simulink model "gm_ZynqBF_2tx_fpga"  (R2018b)
settings: Solver=FixedStepDiscrete  StartTime=0.0  StopTime=10.0  FixedStep=(1/420e3)/128  RelTol=1e-3
undefined symbols (not defined in the file or in its folder): a, b, c
libraries: hdlsllib x873, simulink x349
(part 38 of 40)

== system gm_ZynqBF_2tx_fpga/channel_estimator/peakdetect_ch1/correlator1/rx_ram_q_instance21/get_bit ==
  u : Inport  OutDataTypeStr=fixdt(0, 64, 0)  PortDimensions=1  SampleTime=1.86011904761905e-08
  ind : Inport  Port=2  OutDataTypeStr=fixdt(0, 9, 0)  PortDimensions=1  SampleTime=1.86011904761905e-08
  get_bit : MATLAB Function  TreatAsAtomicUnit=on
  y : Outport
  wires:
  get_bit/1(y) -> y/1
  ind/1 -> get_bit/2(ind)
  u/1 -> get_bit/1(u)

== system gm_ZynqBF_2tx_fpga/channel_estimator/peakdetect_ch1/correlator1/rx_ram_q_instance22/get_bit ==
  u : Inport  OutDataTypeStr=fixdt(0, 64, 0)  PortDimensions=1  SampleTime=1.86011904761905e-08
  ind : Inport  Port=2  OutDataTypeStr=fixdt(0, 9, 0)  PortDimensions=1  SampleTime=1.86011904761905e-08
  get_bit : MATLAB Function  TreatAsAtomicUnit=on
  y : Outport
  wires:
  get_bit/1(y) -> y/1
  ind/1 -> get_bit/2(ind)
  u/1 -> get_bit/1(u)

== system gm_ZynqBF_2tx_fpga/channel_estimator/peakdetect_ch1/correlator1/rx_ram_q_instance23/get_bit ==
  u : Inport  OutDataTypeStr=fixdt(0, 64, 0)  PortDimensions=1  SampleTime=1.86011904761905e-08
  ind : Inport  Port=2  OutDataTypeStr=fixdt(0, 9, 0)  PortDimensions=1  SampleTime=1.86011904761905e-08
  get_bit : MATLAB Function  TreatAsAtomicUnit=on
  y : Outport
  wires:
  get_bit/1(y) -> y/1
  ind/1 -> get_bit/2(ind)
  u/1 -> get_bit/1(u)

== system gm_ZynqBF_2tx_fpga/channel_estimator/peakdetect_ch1/correlator1/rx_ram_q_instance24/get_bit ==
  u : Inport  OutDataTypeStr=fixdt(0, 64, 0)  PortDimensions=1  SampleTime=1.86011904761905e-08
  ind : Inport  Port=2  OutDataTypeStr=fixdt(0, 9, 0)  PortDimensions=1  SampleTime=1.86011904761905e-08
  get_bit : MATLAB Function  TreatAsAtomicUnit=on
  y : Outport
  wires:
  get_bit/1(y) -> y/1
  ind/1 -> get_bit/2(ind)
  u/1 -> get_bit/1(u)

== system gm_ZynqBF_2tx_fpga/channel_estimator/peakdetect_ch1/correlator1/rx_ram_q_instance25/get_bit ==
  u : Inport  OutDataTypeStr=fixdt(0, 64, 0)  PortDimensions=1  SampleTime=1.86011904761905e-08
  ind : Inport  Port=2  OutDataTypeStr=fixdt(0, 9, 0)  PortDimensions=1  SampleTime=1.86011904761905e-08
  get_bit : MATLAB Function  TreatAsAtomicUnit=on
  y : Outport
  wires:
  get_bit/1(y) -> y/1
  ind/1 -> get_bit/2(ind)
  u/1 -> get_bit/1(u)

== system gm_ZynqBF_2tx_fpga/channel_estimator/peakdetect_ch1/correlator1/rx_ram_q_instance26/get_bit ==
  u : Inport  OutDataTypeStr=fixdt(0, 64, 0)  PortDimensions=1  SampleTime=1.86011904761905e-08
  ind : Inport  Port=2  OutDataTypeStr=fixdt(0, 9, 0)  PortDimensions=1  SampleTime=1.86011904761905e-08
  get_bit : MATLAB Function  TreatAsAtomicUnit=on
  y : Outport
  wires:
  get_bit/1(y) -> y/1
  ind/1 -> get_bit/2(ind)
  u/1 -> get_bit/1(u)

== system gm_ZynqBF_2tx_fpga/channel_estimator/peakdetect_ch1/correlator1/rx_ram_q_instance27/get_bit ==
  u : Inport  OutDataTypeStr=fixdt(0, 64, 0)  PortDimensions=1  SampleTime=1.86011904761905e-08
  ind : Inport  Port=2  OutDataTypeStr=fixdt(0, 9, 0)  PortDimensions=1  SampleTime=1.86011904761905e-08
  get_bit : MATLAB Function  TreatAsAtomicUnit=on
  y : Outport
  wires:
  get_bit/1(y) -> y/1
  ind/1 -> get_bit/2(ind)
  u/1 -> get_bit/1(u)

== system gm_ZynqBF_2tx_fpga/channel_estimator/peakdetect_ch1/correlator1/rx_ram_q_instance28/get_bit ==
  u : Inport  OutDataTypeStr=fixdt(0, 64, 0)  PortDimensions=1  SampleTime=1.86011904761905e-08
  ind : Inport  Port=2  OutDataTypeStr=fixdt(0, 9, 0)  PortDimensions=1  SampleTime=1.86011904761905e-08
  get_bit : MATLAB Function  TreatAsAtomicUnit=on
  y : Outport
  wires:
  get_bit/1(y) -> y/1
  ind/1 -> get_bit/2(ind)
  u/1 -> get_bit/1(u)

== system gm_ZynqBF_2tx_fpga/channel_estimator/peakdetect_ch1/correlator1/rx_ram_q_instance29/get_bit ==
  u : Inport  OutDataTypeStr=fixdt(0, 64, 0)  PortDimensions=1  SampleTime=1.86011904761905e-08
  ind : Inport  Port=2  OutDataTypeStr=fixdt(0, 9, 0)  PortDimensions=1  SampleTime=1.86011904761905e-08
  get_bit : MATLAB Function  TreatAsAtomicUnit=on
  y : Outport
  wires:
  get_bit/1(y) -> y/1
  ind/1 -> get_bit/2(ind)
  u/1 -> get_bit/1(u)

== system gm_ZynqBF_2tx_fpga/channel_estimator/peakdetect_ch1/correlator1/rx_ram_q_instance3/get_bit ==
  u : Inport  OutDataTypeStr=fixdt(0, 64, 0)  PortDimensions=1  SampleTime=1.86011904761905e-08
  ind : Inport  Port=2  OutDataTypeStr=fixdt(0, 9, 0)  PortDimensions=1  SampleTime=1.86011904761905e-08
  get_bit : MATLAB Function  TreatAsAtomicUnit=on
  y : Outport
  wires:
  get_bit/1(y) -> y/1
  ind/1 -> get_bit/2(ind)
  u/1 -> get_bit/1(u)

== system gm_ZynqBF_2tx_fpga/channel_estimator/peakdetect_ch1/correlator1/rx_ram_q_instance30/get_bit ==
  u : Inport  OutDataTypeStr=fixdt(0, 64, 0)  PortDimensions=1  SampleTime=1.86011904761905e-08
  ind : Inport  Port=2  OutDataTypeStr=fixdt(0, 9, 0)  PortDimensions=1  SampleTime=1.86011904761905e-08
  get_bit : MATLAB Function  TreatAsAtomicUnit=on
  y : Outport
  wires:
  get_bit/1(y) -> y/1
  ind/1 -> get_bit/2(ind)
  u/1 -> get_bit/1(u)

== system gm_ZynqBF_2tx_fpga/channel_estimator/peakdetect_ch1/correlator1/rx_ram_q_instance31/get_bit ==
  u : Inport  OutDataTypeStr=fixdt(0, 64, 0)  PortDimensions=1  SampleTime=1.86011904761905e-08
  ind : Inport  Port=2  OutDataTypeStr=fixdt(0, 9, 0)  PortDimensions=1  SampleTime=1.86011904761905e-08
  get_bit : MATLAB Function  TreatAsAtomicUnit=on
  y : Outport
  wires:
  get_bit/1(y) -> y/1
  ind/1 -> get_bit/2(ind)
  u/1 -> get_bit/1(u)

== system gm_ZynqBF_2tx_fpga/channel_estimator/peakdetect_ch1/correlator1/rx_ram_q_instance32/get_bit ==
  u : Inport  OutDataTypeStr=fixdt(0, 64, 0)  PortDimensions=1  SampleTime=1.86011904761905e-08
  ind : Inport  Port=2  OutDataTypeStr=fixdt(0, 9, 0)  PortDimensions=1  SampleTime=1.86011904761905e-08
  get_bit : MATLAB Function  TreatAsAtomicUnit=on
  y : Outport
  wires:
  get_bit/1(y) -> y/1
  ind/1 -> get_bit/2(ind)
  u/1 -> get_bit/1(u)

== system gm_ZynqBF_2tx_fpga/channel_estimator/peakdetect_ch1/correlator1/rx_ram_q_instance33/get_bit ==
  u : Inport  OutDataTypeStr=fixdt(0, 64, 0)  PortDimensions=1  SampleTime=1.86011904761905e-08
  ind : Inport  Port=2  OutDataTypeStr=fixdt(0, 9, 0)  PortDimensions=1  SampleTime=1.86011904761905e-08
  get_bit : MATLAB Function  TreatAsAtomicUnit=on
  y : Outport
  wires:
  get_bit/1(y) -> y/1
  ind/1 -> get_bit/2(ind)
  u/1 -> get_bit/1(u)

== system gm_ZynqBF_2tx_fpga/channel_estimator/peakdetect_ch1/correlator1/rx_ram_q_instance34/get_bit ==
  u : Inport  OutDataTypeStr=fixdt(0, 64, 0)  PortDimensions=1  SampleTime=1.86011904761905e-08
  ind : Inport  Port=2  OutDataTypeStr=fixdt(0, 9, 0)  PortDimensions=1  SampleTime=1.86011904761905e-08
  get_bit : MATLAB Function  TreatAsAtomicUnit=on
  y : Outport
  wires:
  get_bit/1(y) -> y/1
  ind/1 -> get_bit/2(ind)
  u/1 -> get_bit/1(u)

== system gm_ZynqBF_2tx_fpga/channel_estimator/peakdetect_ch1/correlator1/rx_ram_q_instance35/get_bit ==
  u : Inport  OutDataTypeStr=fixdt(0, 64, 0)  PortDimensions=1  SampleTime=1.86011904761905e-08
  ind : Inport  Port=2  OutDataTypeStr=fixdt(0, 9, 0)  PortDimensions=1  SampleTime=1.86011904761905e-08
  get_bit : MATLAB Function  TreatAsAtomicUnit=on
  y : Outport
  wires:
  get_bit/1(y) -> y/1
  ind/1 -> get_bit/2(ind)
  u/1 -> get_bit/1(u)

== system gm_ZynqBF_2tx_fpga/channel_estimator/peakdetect_ch1/correlator1/rx_ram_q_instance36/get_bit ==
  u : Inport  OutDataTypeStr=fixdt(0, 64, 0)  PortDimensions=1  SampleTime=1.86011904761905e-08
  ind : Inport  Port=2  OutDataTypeStr=fixdt(0, 9, 0)  PortDimensions=1  SampleTime=1.86011904761905e-08
  get_bit : MATLAB Function  TreatAsAtomicUnit=on
  y : Outport
  wires:
  get_bit/1(y) -> y/1
  ind/1 -> get_bit/2(ind)
  u/1 -> get_bit/1(u)

== system gm_ZynqBF_2tx_fpga/channel_estimator/peakdetect_ch1/correlator1/rx_ram_q_instance37/get_bit ==
  u : Inport  OutDataTypeStr=fixdt(0, 64, 0)  PortDimensions=1  SampleTime=1.86011904761905e-08
  ind : Inport  Port=2  OutDataTypeStr=fixdt(0, 9, 0)  PortDimensions=1  SampleTime=1.86011904761905e-08
  get_bit : MATLAB Function  TreatAsAtomicUnit=on
  y : Outport
  wires:
  get_bit/1(y) -> y/1
  ind/1 -> get_bit/2(ind)
  u/1 -> get_bit/1(u)

== system gm_ZynqBF_2tx_fpga/channel_estimator/peakdetect_ch1/correlator1/rx_ram_q_instance38/get_bit ==
  u : Inport  OutDataTypeStr=fixdt(0, 64, 0)  PortDimensions=1  SampleTime=1.86011904761905e-08
  ind : Inport  Port=2  OutDataTypeStr=fixdt(0, 9, 0)  PortDimensions=1  SampleTime=1.86011904761905e-08
  get_bit : MATLAB Function  TreatAsAtomicUnit=on
  y : Outport
  wires:
  get_bit/1(y) -> y/1
  ind/1 -> get_bit/2(ind)
  u/1 -> get_bit/1(u)

== system gm_ZynqBF_2tx_fpga/channel_estimator/peakdetect_ch1/correlator1/rx_ram_q_instance39/get_bit ==
  u : Inport  OutDataTypeStr=fixdt(0, 64, 0)  PortDimensions=1  SampleTime=1.86011904761905e-08
  ind : Inport  Port=2  OutDataTypeStr=fixdt(0, 9, 0)  PortDimensions=1  SampleTime=1.86011904761905e-08
  get_bit : MATLAB Function  TreatAsAtomicUnit=on
  y : Outport
  wires:
  get_bit/1(y) -> y/1
  ind/1 -> get_bit/2(ind)
  u/1 -> get_bit/1(u)

== system gm_ZynqBF_2tx_fpga/channel_estimator/peakdetect_ch1/correlator1/rx_ram_q_instance4/get_bit ==
  u : Inport  OutDataTypeStr=fixdt(0, 64, 0)  PortDimensions=1  SampleTime=1.86011904761905e-08
  ind : Inport  Port=2  OutDataTypeStr=fixdt(0, 9, 0)  PortDimensions=1  SampleTime=1.86011904761905e-08
  get_bit : MATLAB Function  TreatAsAtomicUnit=on
  y : Outport
  wires:
  get_bit/1(y) -> y/1
  ind/1 -> get_bit/2(ind)
  u/1 -> get_bit/1(u)

== system gm_ZynqBF_2tx_fpga/channel_estimator/peakdetect_ch1/correlator1/rx_ram_q_instance40/get_bit ==
  u : Inport  OutDataTypeStr=fixdt(0, 64, 0)  PortDimensions=1  SampleTime=1.86011904761905e-08
  ind : Inport  Port=2  OutDataTypeStr=fixdt(0, 9, 0)  PortDimensions=1  SampleTime=1.86011904761905e-08
  get_bit : MATLAB Function  TreatAsAtomicUnit=on
  y : Outport
  wires:
  get_bit/1(y) -> y/1
  ind/1 -> get_bit/2(ind)
  u/1 -> get_bit/1(u)

== system gm_ZynqBF_2tx_fpga/channel_estimator/peakdetect_ch1/correlator1/rx_ram_q_instance41/get_bit ==
  u : Inport  OutDataTypeStr=fixdt(0, 64, 0)  PortDimensions=1  SampleTime=1.86011904761905e-08
  ind : Inport  Port=2  OutDataTypeStr=fixdt(0, 9, 0)  PortDimensions=1  SampleTime=1.86011904761905e-08
  get_bit : MATLAB Function  TreatAsAtomicUnit=on
  y : Outport
  wires:
  get_bit/1(y) -> y/1
  ind/1 -> get_bit/2(ind)
  u/1 -> get_bit/1(u)

== system gm_ZynqBF_2tx_fpga/channel_estimator/peakdetect_ch1/correlator1/rx_ram_q_instance42/get_bit ==
  u : Inport  OutDataTypeStr=fixdt(0, 64, 0)  PortDimensions=1  SampleTime=1.86011904761905e-08
  ind : Inport  Port=2  OutDataTypeStr=fixdt(0, 9, 0)  PortDimensions=1  SampleTime=1.86011904761905e-08
  get_bit : MATLAB Function  TreatAsAtomicUnit=on
  y : Outport
  wires:
  get_bit/1(y) -> y/1
  ind/1 -> get_bit/2(ind)
  u/1 -> get_bit/1(u)

== system gm_ZynqBF_2tx_fpga/channel_estimator/peakdetect_ch1/correlator1/rx_ram_q_instance43/get_bit ==
  u : Inport  OutDataTypeStr=fixdt(0, 64, 0)  PortDimensions=1  SampleTime=1.86011904761905e-08
  ind : Inport  Port=2  OutDataTypeStr=fixdt(0, 9, 0)  PortDimensions=1  SampleTime=1.86011904761905e-08
  get_bit : MATLAB Function  TreatAsAtomicUnit=on
  y : Outport
  wires:
  get_bit/1(y) -> y/1
  ind/1 -> get_bit/2(ind)
  u/1 -> get_bit/1(u)

== system gm_ZynqBF_2tx_fpga/channel_estimator/peakdetect_ch1/correlator1/rx_ram_q_instance44/get_bit ==
  u : Inport  OutDataTypeStr=fixdt(0, 64, 0)  PortDimensions=1  SampleTime=1.86011904761905e-08
  ind : Inport  Port=2  OutDataTypeStr=fixdt(0, 9, 0)  PortDimensions=1  SampleTime=1.86011904761905e-08
  get_bit : MATLAB Function  TreatAsAtomicUnit=on
  y : Outport
  wires:
  get_bit/1(y) -> y/1
  ind/1 -> get_bit/2(ind)
  u/1 -> get_bit/1(u)

== system gm_ZynqBF_2tx_fpga/channel_estimator/peakdetect_ch1/correlator1/rx_ram_q_instance45/get_bit ==
  u : Inport  OutDataTypeStr=fixdt(0, 64, 0)  PortDimensions=1  SampleTime=1.86011904761905e-08
  ind : Inport  Port=2  OutDataTypeStr=fixdt(0, 9, 0)  PortDimensions=1  SampleTime=1.86011904761905e-08
  get_bit : MATLAB Function  TreatAsAtomicUnit=on
  y : Outport
  wires:
  get_bit/1(y) -> y/1
  ind/1 -> get_bit/2(ind)
  u/1 -> get_bit/1(u)

== system gm_ZynqBF_2tx_fpga/channel_estimator/peakdetect_ch1/correlator1/rx_ram_q_instance46/get_bit ==
  u : Inport  OutDataTypeStr=fixdt(0, 64, 0)  PortDimensions=1  SampleTime=1.86011904761905e-08
  ind : Inport  Port=2  OutDataTypeStr=fixdt(0, 9, 0)  PortDimensions=1  SampleTime=1.86011904761905e-08
  get_bit : MATLAB Function  TreatAsAtomicUnit=on
  y : Outport
  wires:
  get_bit/1(y) -> y/1
  ind/1 -> get_bit/2(ind)
  u/1 -> get_bit/1(u)

== system gm_ZynqBF_2tx_fpga/channel_estimator/peakdetect_ch1/correlator1/rx_ram_q_instance47/get_bit ==
  u : Inport  OutDataTypeStr=fixdt(0, 64, 0)  PortDimensions=1  SampleTime=1.86011904761905e-08
  ind : Inport  Port=2  OutDataTypeStr=fixdt(0, 9, 0)  PortDimensions=1  SampleTime=1.86011904761905e-08
  get_bit : MATLAB Function  TreatAsAtomicUnit=on
  y : Outport
  wires:
  get_bit/1(y) -> y/1
  ind/1 -> get_bit/2(ind)
  u/1 -> get_bit/1(u)

== system gm_ZynqBF_2tx_fpga/channel_estimator/peakdetect_ch1/correlator1/rx_ram_q_instance48/get_bit ==
  u : Inport  OutDataTypeStr=fixdt(0, 64, 0)  PortDimensions=1  SampleTime=1.86011904761905e-08
  ind : Inport  Port=2  OutDataTypeStr=fixdt(0, 9, 0)  PortDimensions=1  SampleTime=1.86011904761905e-08
  get_bit : MATLAB Function  TreatAsAtomicUnit=on
  y : Outport
  wires:
  get_bit/1(y) -> y/1
  ind/1 -> get_bit/2(ind)
  u/1 -> get_bit/1(u)

== system gm_ZynqBF_2tx_fpga/channel_estimator/peakdetect_ch1/correlator1/rx_ram_q_instance49/get_bit ==
  u : Inport  OutDataTypeStr=fixdt(0, 64, 0)  PortDimensions=1  SampleTime=1.86011904761905e-08
  ind : Inport  Port=2  OutDataTypeStr=fixdt(0, 9, 0)  PortDimensions=1  SampleTime=1.86011904761905e-08
  get_bit : MATLAB Function  TreatAsAtomicUnit=on
  y : Outport
  wires:
  get_bit/1(y) -> y/1
  ind/1 -> get_bit/2(ind)
  u/1 -> get_bit/1(u)

== system gm_ZynqBF_2tx_fpga/channel_estimator/peakdetect_ch1/correlator1/rx_ram_q_instance5/get_bit ==
  u : Inport  OutDataTypeStr=fixdt(0, 64, 0)  PortDimensions=1  SampleTime=1.86011904761905e-08
  ind : Inport  Port=2  OutDataTypeStr=fixdt(0, 9, 0)  PortDimensions=1  SampleTime=1.86011904761905e-08
  get_bit : MATLAB Function  TreatAsAtomicUnit=on
  y : Outport
  wires:
  get_bit/1(y) -> y/1
  ind/1 -> get_bit/2(ind)
  u/1 -> get_bit/1(u)

== system gm_ZynqBF_2tx_fpga/channel_estimator/peakdetect_ch1/correlator1/rx_ram_q_instance50/get_bit ==
  u : Inport  OutDataTypeStr=fixdt(0, 64, 0)  PortDimensions=1  SampleTime=1.86011904761905e-08
  ind : Inport  Port=2  OutDataTypeStr=fixdt(0, 9, 0)  PortDimensions=1  SampleTime=1.86011904761905e-08
  get_bit : MATLAB Function  TreatAsAtomicUnit=on
  y : Outport
  wires:
  get_bit/1(y) -> y/1
  ind/1 -> get_bit/2(ind)
  u/1 -> get_bit/1(u)

== system gm_ZynqBF_2tx_fpga/channel_estimator/peakdetect_ch1/correlator1/rx_ram_q_instance51/get_bit ==
  u : Inport  OutDataTypeStr=fixdt(0, 64, 0)  PortDimensions=1  SampleTime=1.86011904761905e-08
  ind : Inport  Port=2  OutDataTypeStr=fixdt(0, 9, 0)  PortDimensions=1  SampleTime=1.86011904761905e-08
  get_bit : MATLAB Function  TreatAsAtomicUnit=on
  y : Outport
  wires:
  get_bit/1(y) -> y/1
  ind/1 -> get_bit/2(ind)
  u/1 -> get_bit/1(u)

== system gm_ZynqBF_2tx_fpga/channel_estimator/peakdetect_ch1/correlator1/rx_ram_q_instance52/get_bit ==
  u : Inport  OutDataTypeStr=fixdt(0, 64, 0)  PortDimensions=1  SampleTime=1.86011904761905e-08
  ind : Inport  Port=2  OutDataTypeStr=fixdt(0, 9, 0)  PortDimensions=1  SampleTime=1.86011904761905e-08
  get_bit : MATLAB Function  TreatAsAtomicUnit=on
  y : Outport
  wires:
  get_bit/1(y) -> y/1
  ind/1 -> get_bit/2(ind)
  u/1 -> get_bit/1(u)

== system gm_ZynqBF_2tx_fpga/channel_estimator/peakdetect_ch1/correlator1/rx_ram_q_instance53/get_bit ==
  u : Inport  OutDataTypeStr=fixdt(0, 64, 0)  PortDimensions=1  SampleTime=1.86011904761905e-08
  ind : Inport  Port=2  OutDataTypeStr=fixdt(0, 9, 0)  PortDimensions=1  SampleTime=1.86011904761905e-08
  get_bit : MATLAB Function  TreatAsAtomicUnit=on
  y : Outport
  wires:
  get_bit/1(y) -> y/1
  ind/1 -> get_bit/2(ind)
  u/1 -> get_bit/1(u)

== system gm_ZynqBF_2tx_fpga/channel_estimator/peakdetect_ch1/correlator1/rx_ram_q_instance54/get_bit ==
  u : Inport  OutDataTypeStr=fixdt(0, 64, 0)  PortDimensions=1  SampleTime=1.86011904761905e-08
  ind : Inport  Port=2  OutDataTypeStr=fixdt(0, 9, 0)  PortDimensions=1  SampleTime=1.86011904761905e-08
  get_bit : MATLAB Function  TreatAsAtomicUnit=on
  y : Outport
  wires:
  get_bit/1(y) -> y/1
  ind/1 -> get_bit/2(ind)
  u/1 -> get_bit/1(u)

== system gm_ZynqBF_2tx_fpga/channel_estimator/peakdetect_ch1/correlator1/rx_ram_q_instance55/get_bit ==
  u : Inport  OutDataTypeStr=fixdt(0, 64, 0)  PortDimensions=1  SampleTime=1.86011904761905e-08
  ind : Inport  Port=2  OutDataTypeStr=fixdt(0, 9, 0)  PortDimensions=1  SampleTime=1.86011904761905e-08
  get_bit : MATLAB Function  TreatAsAtomicUnit=on
  y : Outport
  wires:
  get_bit/1(y) -> y/1
  ind/1 -> get_bit/2(ind)
  u/1 -> get_bit/1(u)

== system gm_ZynqBF_2tx_fpga/channel_estimator/peakdetect_ch1/correlator1/rx_ram_q_instance56/get_bit ==
  u : Inport  OutDataTypeStr=fixdt(0, 64, 0)  PortDimensions=1  SampleTime=1.86011904761905e-08
  ind : Inport  Port=2  OutDataTypeStr=fixdt(0, 9, 0)  PortDimensions=1  SampleTime=1.86011904761905e-08
  get_bit : MATLAB Function  TreatAsAtomicUnit=on
  y : Outport
  wires:
  get_bit/1(y) -> y/1
  ind/1 -> get_bit/2(ind)
  u/1 -> get_bit/1(u)

== system gm_ZynqBF_2tx_fpga/channel_estimator/peakdetect_ch1/correlator1/rx_ram_q_instance57/get_bit ==
  u : Inport  OutDataTypeStr=fixdt(0, 64, 0)  PortDimensions=1  SampleTime=1.86011904761905e-08
  ind : Inport  Port=2  OutDataTypeStr=fixdt(0, 9, 0)  PortDimensions=1  SampleTime=1.86011904761905e-08
  get_bit : MATLAB Function  TreatAsAtomicUnit=on
  y : Outport
  wires:
  get_bit/1(y) -> y/1
  ind/1 -> get_bit/2(ind)
  u/1 -> get_bit/1(u)

== system gm_ZynqBF_2tx_fpga/channel_estimator/peakdetect_ch1/correlator1/rx_ram_q_instance58/get_bit ==
  u : Inport  OutDataTypeStr=fixdt(0, 64, 0)  PortDimensions=1  SampleTime=1.86011904761905e-08
  ind : Inport  Port=2  OutDataTypeStr=fixdt(0, 9, 0)  PortDimensions=1  SampleTime=1.86011904761905e-08
  get_bit : MATLAB Function  TreatAsAtomicUnit=on
  y : Outport
  wires:
  get_bit/1(y) -> y/1
  ind/1 -> get_bit/2(ind)
  u/1 -> get_bit/1(u)

== system gm_ZynqBF_2tx_fpga/channel_estimator/peakdetect_ch1/correlator1/rx_ram_q_instance59/get_bit ==
  u : Inport  OutDataTypeStr=fixdt(0, 64, 0)  PortDimensions=1  SampleTime=1.86011904761905e-08
  ind : Inport  Port=2  OutDataTypeStr=fixdt(0, 9, 0)  PortDimensions=1  SampleTime=1.86011904761905e-08
  get_bit : MATLAB Function  TreatAsAtomicUnit=on
  y : Outport
  wires:
  get_bit/1(y) -> y/1
  ind/1 -> get_bit/2(ind)
  u/1 -> get_bit/1(u)

== system gm_ZynqBF_2tx_fpga/channel_estimator/peakdetect_ch1/correlator1/rx_ram_q_instance6/get_bit ==
  u : Inport  OutDataTypeStr=fixdt(0, 64, 0)  PortDimensions=1  SampleTime=1.86011904761905e-08
  ind : Inport  Port=2  OutDataTypeStr=fixdt(0, 9, 0)  PortDimensions=1  SampleTime=1.86011904761905e-08
  get_bit : MATLAB Function  TreatAsAtomicUnit=on
  y : Outport
  wires:
  get_bit/1(y) -> y/1
  ind/1 -> get_bit/2(ind)
  u/1 -> get_bit/1(u)

== system gm_ZynqBF_2tx_fpga/channel_estimator/peakdetect_ch1/correlator1/rx_ram_q_instance60/get_bit ==
  u : Inport  OutDataTypeStr=fixdt(0, 64, 0)  PortDimensions=1  SampleTime=1.86011904761905e-08
  ind : Inport  Port=2  OutDataTypeStr=fixdt(0, 9, 0)  PortDimensions=1  SampleTime=1.86011904761905e-08
  get_bit : MATLAB Function  TreatAsAtomicUnit=on
  y : Outport
  wires:
  get_bit/1(y) -> y/1
  ind/1 -> get_bit/2(ind)
  u/1 -> get_bit/1(u)

== system gm_ZynqBF_2tx_fpga/channel_estimator/peakdetect_ch1/correlator1/rx_ram_q_instance61/get_bit ==
  u : Inport  OutDataTypeStr=fixdt(0, 64, 0)  PortDimensions=1  SampleTime=1.86011904761905e-08
  ind : Inport  Port=2  OutDataTypeStr=fixdt(0, 9, 0)  PortDimensions=1  SampleTime=1.86011904761905e-08
  get_bit : MATLAB Function  TreatAsAtomicUnit=on
  y : Outport
  wires:
  get_bit/1(y) -> y/1
  ind/1 -> get_bit/2(ind)
  u/1 -> get_bit/1(u)

== system gm_ZynqBF_2tx_fpga/channel_estimator/peakdetect_ch1/correlator1/rx_ram_q_instance62/get_bit ==
  u : Inport  OutDataTypeStr=fixdt(0, 64, 0)  PortDimensions=1  SampleTime=1.86011904761905e-08
  ind : Inport  Port=2  OutDataTypeStr=fixdt(0, 9, 0)  PortDimensions=1  SampleTime=1.86011904761905e-08
  get_bit : MATLAB Function  TreatAsAtomicUnit=on
  y : Outport
  wires:
  get_bit/1(y) -> y/1
  ind/1 -> get_bit/2(ind)
  u/1 -> get_bit/1(u)

== system gm_ZynqBF_2tx_fpga/channel_estimator/peakdetect_ch1/correlator1/rx_ram_q_instance63/get_bit ==
  u : Inport  OutDataTypeStr=fixdt(0, 64, 0)  PortDimensions=1  SampleTime=1.86011904761905e-08
  ind : Inport  Port=2  OutDataTypeStr=fixdt(0, 9, 0)  PortDimensions=1  SampleTime=1.86011904761905e-08
  get_bit : MATLAB Function  TreatAsAtomicUnit=on
  y : Outport
  wires:
  get_bit/1(y) -> y/1
  ind/1 -> get_bit/2(ind)
  u/1 -> get_bit/1(u)

== system gm_ZynqBF_2tx_fpga/channel_estimator/peakdetect_ch1/correlator1/rx_ram_q_instance64/get_bit ==
  u : Inport  OutDataTypeStr=fixdt(0, 64, 0)  PortDimensions=1  SampleTime=1.86011904761905e-08
  ind : Inport  Port=2  OutDataTypeStr=fixdt(0, 9, 0)  PortDimensions=1  SampleTime=1.86011904761905e-08
  get_bit : MATLAB Function  TreatAsAtomicUnit=on
  y : Outport
  wires:
  get_bit/1(y) -> y/1
  ind/1 -> get_bit/2(ind)
  u/1 -> get_bit/1(u)

== system gm_ZynqBF_2tx_fpga/channel_estimator/peakdetect_ch1/correlator1/rx_ram_q_instance7/get_bit ==
  u : Inport  OutDataTypeStr=fixdt(0, 64, 0)  PortDimensions=1  SampleTime=1.86011904761905e-08
  ind : Inport  Port=2  OutDataTypeStr=fixdt(0, 9, 0)  PortDimensions=1  SampleTime=1.86011904761905e-08
  get_bit : MATLAB Function  TreatAsAtomicUnit=on
  y : Outport
  wires:
  get_bit/1(y) -> y/1
  ind/1 -> get_bit/2(ind)
  u/1 -> get_bit/1(u)

== system gm_ZynqBF_2tx_fpga/channel_estimator/peakdetect_ch1/correlator1/rx_ram_q_instance8/get_bit ==
  u : Inport  OutDataTypeStr=fixdt(0, 64, 0)  PortDimensions=1  SampleTime=1.86011904761905e-08
  ind : Inport  Port=2  OutDataTypeStr=fixdt(0, 9, 0)  PortDimensions=1  SampleTime=1.86011904761905e-08
  get_bit : MATLAB Function  TreatAsAtomicUnit=on
  y : Outport
  wires:
  get_bit/1(y) -> y/1
  ind/1 -> get_bit/2(ind)
  u/1 -> get_bit/1(u)

== system gm_ZynqBF_2tx_fpga/channel_estimator/peakdetect_ch1/correlator1/rx_ram_q_instance9/get_bit ==
  u : Inport  OutDataTypeStr=fixdt(0, 64, 0)  PortDimensions=1  SampleTime=1.86011904761905e-08
  ind : Inport  Port=2  OutDataTypeStr=fixdt(0, 9, 0)  PortDimensions=1  SampleTime=1.86011904761905e-08
  get_bit : MATLAB Function  TreatAsAtomicUnit=on
  y : Outport
  wires:
  get_bit/1(y) -> y/1
  ind/1 -> get_bit/2(ind)
  u/1 -> get_bit/1(u)

== system gm_ZynqBF_2tx_fpga/channel_estimator/peakdetect_ch2/correlator2/rx_ram_i_instance1/get_bit ==
  u : Inport  OutDataTypeStr=fixdt(0, 64, 0)  PortDimensions=1  SampleTime=1.86011904761905e-08
  ind : Inport  Port=2  OutDataTypeStr=fixdt(0, 9, 0)  PortDimensions=1  SampleTime=1.86011904761905e-08
  get_bit : MATLAB Function  TreatAsAtomicUnit=on
  y : Outport
  wires:
  get_bit/1(y) -> y/1
  ind/1 -> get_bit/2(ind)
  u/1 -> get_bit/1(u)

== system gm_ZynqBF_2tx_fpga/channel_estimator/peakdetect_ch2/correlator2/rx_ram_i_instance10/get_bit ==
  u : Inport  OutDataTypeStr=fixdt(0, 64, 0)  PortDimensions=1  SampleTime=1.86011904761905e-08
  ind : Inport  Port=2  OutDataTypeStr=fixdt(0, 9, 0)  PortDimensions=1  SampleTime=1.86011904761905e-08
  get_bit : MATLAB Function  TreatAsAtomicUnit=on
  y : Outport
  wires:
  get_bit/1(y) -> y/1
  ind/1 -> get_bit/2(ind)
  u/1 -> get_bit/1(u)

== system gm_ZynqBF_2tx_fpga/channel_estimator/peakdetect_ch2/correlator2/rx_ram_i_instance11/get_bit ==
  u : Inport  OutDataTypeStr=fixdt(0, 64, 0)  PortDimensions=1  SampleTime=1.86011904761905e-08
  ind : Inport  Port=2  OutDataTypeStr=fixdt(0, 9, 0)  PortDimensions=1  SampleTime=1.86011904761905e-08
  get_bit : MATLAB Function  TreatAsAtomicUnit=on
  y : Outport
  wires:
  get_bit/1(y) -> y/1
  ind/1 -> get_bit/2(ind)
  u/1 -> get_bit/1(u)

== system gm_ZynqBF_2tx_fpga/channel_estimator/peakdetect_ch2/correlator2/rx_ram_i_instance12/get_bit ==
  u : Inport  OutDataTypeStr=fixdt(0, 64, 0)  PortDimensions=1  SampleTime=1.86011904761905e-08
  ind : Inport  Port=2  OutDataTypeStr=fixdt(0, 9, 0)  PortDimensions=1  SampleTime=1.86011904761905e-08
  get_bit : MATLAB Function  TreatAsAtomicUnit=on
  y : Outport
  wires:
  get_bit/1(y) -> y/1
  ind/1 -> get_bit/2(ind)
  u/1 -> get_bit/1(u)

== system gm_ZynqBF_2tx_fpga/channel_estimator/peakdetect_ch2/correlator2/rx_ram_i_instance13/get_bit ==
  u : Inport  OutDataTypeStr=fixdt(0, 64, 0)  PortDimensions=1  SampleTime=1.86011904761905e-08
  ind : Inport  Port=2  OutDataTypeStr=fixdt(0, 9, 0)  PortDimensions=1  SampleTime=1.86011904761905e-08
  get_bit : MATLAB Function  TreatAsAtomicUnit=on
  y : Outport
  wires:
  get_bit/1(y) -> y/1
  ind/1 -> get_bit/2(ind)
  u/1 -> get_bit/1(u)

== system gm_ZynqBF_2tx_fpga/channel_estimator/peakdetect_ch2/correlator2/rx_ram_i_instance14/get_bit ==
  u : Inport  OutDataTypeStr=fixdt(0, 64, 0)  PortDimensions=1  SampleTime=1.86011904761905e-08
  ind : Inport  Port=2  OutDataTypeStr=fixdt(0, 9, 0)  PortDimensions=1  SampleTime=1.86011904761905e-08
  get_bit : MATLAB Function  TreatAsAtomicUnit=on
  y : Outport
  wires:
  get_bit/1(y) -> y/1
  ind/1 -> get_bit/2(ind)
  u/1 -> get_bit/1(u)

== system gm_ZynqBF_2tx_fpga/channel_estimator/peakdetect_ch2/correlator2/rx_ram_i_instance15/get_bit ==
  u : Inport  OutDataTypeStr=fixdt(0, 64, 0)  PortDimensions=1  SampleTime=1.86011904761905e-08
  ind : Inport  Port=2  OutDataTypeStr=fixdt(0, 9, 0)  PortDimensions=1  SampleTime=1.86011904761905e-08
  get_bit : MATLAB Function  TreatAsAtomicUnit=on
  y : Outport
  wires:
  get_bit/1(y) -> y/1
  ind/1 -> get_bit/2(ind)
  u/1 -> get_bit/1(u)

== system gm_ZynqBF_2tx_fpga/channel_estimator/peakdetect_ch2/correlator2/rx_ram_i_instance16/get_bit ==
  u : Inport  OutDataTypeStr=fixdt(0, 64, 0)  PortDimensions=1  SampleTime=1.86011904761905e-08
  ind : Inport  Port=2  OutDataTypeStr=fixdt(0, 9, 0)  PortDimensions=1  SampleTime=1.86011904761905e-08
  get_bit : MATLAB Function  TreatAsAtomicUnit=on
  y : Outport
  wires:
  get_bit/1(y) -> y/1
  ind/1 -> get_bit/2(ind)
  u/1 -> get_bit/1(u)

== system gm_ZynqBF_2tx_fpga/channel_estimator/peakdetect_ch2/correlator2/rx_ram_i_instance17/get_bit ==
  u : Inport  OutDataTypeStr=fixdt(0, 64, 0)  PortDimensions=1  SampleTime=1.86011904761905e-08
  ind : Inport  Port=2  OutDataTypeStr=fixdt(0, 9, 0)  PortDimensions=1  SampleTime=1.86011904761905e-08
  get_bit : MATLAB Function  TreatAsAtomicUnit=on
  y : Outport
  wires:
  get_bit/1(y) -> y/1
  ind/1 -> get_bit/2(ind)
  u/1 -> get_bit/1(u)

== system gm_ZynqBF_2tx_fpga/channel_estimator/peakdetect_ch2/correlator2/rx_ram_i_instance18/get_bit ==
  u : Inport  OutDataTypeStr=fixdt(0, 64, 0)  PortDimensions=1  SampleTime=1.86011904761905e-08
  ind : Inport  Port=2  OutDataTypeStr=fixdt(0, 9, 0)  PortDimensions=1  SampleTime=1.86011904761905e-08
  get_bit : MATLAB Function  TreatAsAtomicUnit=on
  y : Outport
  wires:
  get_bit/1(y) -> y/1
  ind/1 -> get_bit/2(ind)
  u/1 -> get_bit/1(u)

== system gm_ZynqBF_2tx_fpga/channel_estimator/peakdetect_ch2/correlator2/rx_ram_i_instance19/get_bit ==
  u : Inport  OutDataTypeStr=fixdt(0, 64, 0)  PortDimensions=1  SampleTime=1.86011904761905e-08
  ind : Inport  Port=2  OutDataTypeStr=fixdt(0, 9, 0)  PortDimensions=1  SampleTime=1.86011904761905e-08
  get_bit : MATLAB Function  TreatAsAtomicUnit=on
  y : Outport
  wires:
  get_bit/1(y) -> y/1
  ind/1 -> get_bit/2(ind)
  u/1 -> get_bit/1(u)

== system gm_ZynqBF_2tx_fpga/channel_estimator/peakdetect_ch2/correlator2/rx_ram_i_instance2/get_bit ==
  u : Inport  OutDataTypeStr=fixdt(0, 64, 0)  PortDimensions=1  SampleTime=1.86011904761905e-08
  ind : Inport  Port=2  OutDataTypeStr=fixdt(0, 9, 0)  PortDimensions=1  SampleTime=1.86011904761905e-08
  get_bit : MATLAB Function  TreatAsAtomicUnit=on
  y : Outport
  wires:
  get_bit/1(y) -> y/1
  ind/1 -> get_bit/2(ind)
  u/1 -> get_bit/1(u)

== system gm_ZynqBF_2tx_fpga/channel_estimator/peakdetect_ch2/correlator2/rx_ram_i_instance20/get_bit ==
  u : Inport  OutDataTypeStr=fixdt(0, 64, 0)  PortDimensions=1  SampleTime=1.86011904761905e-08
  ind : Inport  Port=2  OutDataTypeStr=fixdt(0, 9, 0)  PortDimensions=1  SampleTime=1.86011904761905e-08
  get_bit : MATLAB Function  TreatAsAtomicUnit=on
  y : Outport
  wires:
  get_bit/1(y) -> y/1
  ind/1 -> get_bit/2(ind)
  u/1 -> get_bit/1(u)

== system gm_ZynqBF_2tx_fpga/channel_estimator/peakdetect_ch2/correlator2/rx_ram_i_instance21/get_bit ==
  u : Inport  OutDataTypeStr=fixdt(0, 64, 0)  PortDimensions=1  SampleTime=1.86011904761905e-08
  ind : Inport  Port=2  OutDataTypeStr=fixdt(0, 9, 0)  PortDimensions=1  SampleTime=1.86011904761905e-08
  get_bit : MATLAB Function  TreatAsAtomicUnit=on
  y : Outport
  wires:
  get_bit/1(y) -> y/1
  ind/1 -> get_bit/2(ind)
  u/1 -> get_bit/1(u)

== system gm_ZynqBF_2tx_fpga/channel_estimator/peakdetect_ch2/correlator2/rx_ram_i_instance22/get_bit ==
  u : Inport  OutDataTypeStr=fixdt(0, 64, 0)  PortDimensions=1  SampleTime=1.86011904761905e-08
  ind : Inport  Port=2  OutDataTypeStr=fixdt(0, 9, 0)  PortDimensions=1  SampleTime=1.86011904761905e-08
  get_bit : MATLAB Function  TreatAsAtomicUnit=on
  y : Outport
  wires:
  get_bit/1(y) -> y/1
  ind/1 -> get_bit/2(ind)
  u/1 -> get_bit/1(u)

== system gm_ZynqBF_2tx_fpga/channel_estimator/peakdetect_ch2/correlator2/rx_ram_i_instance23/get_bit ==
  u : Inport  OutDataTypeStr=fixdt(0, 64, 0)  PortDimensions=1  SampleTime=1.86011904761905e-08
  ind : Inport  Port=2  OutDataTypeStr=fixdt(0, 9, 0)  PortDimensions=1  SampleTime=1.86011904761905e-08
  get_bit : MATLAB Function  TreatAsAtomicUnit=on
  y : Outport
  wires:
  get_bit/1(y) -> y/1
  ind/1 -> get_bit/2(ind)
  u/1 -> get_bit/1(u)

== system gm_ZynqBF_2tx_fpga/channel_estimator/peakdetect_ch2/correlator2/rx_ram_i_instance24/get_bit ==
  u : Inport  OutDataTypeStr=fixdt(0, 64, 0)  PortDimensions=1  SampleTime=1.86011904761905e-08
  ind : Inport  Port=2  OutDataTypeStr=fixdt(0, 9, 0)  PortDimensions=1  SampleTime=1.86011904761905e-08
  get_bit : MATLAB Function  TreatAsAtomicUnit=on
  y : Outport
  wires:
  get_bit/1(y) -> y/1
  ind/1 -> get_bit/2(ind)
  u/1 -> get_bit/1(u)

== system gm_ZynqBF_2tx_fpga/channel_estimator/peakdetect_ch2/correlator2/rx_ram_i_instance25/get_bit ==
  u : Inport  OutDataTypeStr=fixdt(0, 64, 0)  PortDimensions=1  SampleTime=1.86011904761905e-08
  ind : Inport  Port=2  OutDataTypeStr=fixdt(0, 9, 0)  PortDimensions=1  SampleTime=1.86011904761905e-08
  get_bit : MATLAB Function  TreatAsAtomicUnit=on
  y : Outport
  wires:
  get_bit/1(y) -> y/1
  ind/1 -> get_bit/2(ind)
  u/1 -> get_bit/1(u)

== system gm_ZynqBF_2tx_fpga/channel_estimator/peakdetect_ch2/correlator2/rx_ram_i_instance26/get_bit ==
  u : Inport  OutDataTypeStr=fixdt(0, 64, 0)  PortDimensions=1  SampleTime=1.86011904761905e-08
  ind : Inport  Port=2  OutDataTypeStr=fixdt(0, 9, 0)  PortDimensions=1  SampleTime=1.86011904761905e-08
  get_bit : MATLAB Function  TreatAsAtomicUnit=on
  y : Outport
  wires:
  get_bit/1(y) -> y/1
  ind/1 -> get_bit/2(ind)
  u/1 -> get_bit/1(u)

== system gm_ZynqBF_2tx_fpga/channel_estimator/peakdetect_ch2/correlator2/rx_ram_i_instance27/get_bit ==
  u : Inport  OutDataTypeStr=fixdt(0, 64, 0)  PortDimensions=1  SampleTime=1.86011904761905e-08
  ind : Inport  Port=2  OutDataTypeStr=fixdt(0, 9, 0)  PortDimensions=1  SampleTime=1.86011904761905e-08
  get_bit : MATLAB Function  TreatAsAtomicUnit=on
  y : Outport
  wires:
  get_bit/1(y) -> y/1
  ind/1 -> get_bit/2(ind)
  u/1 -> get_bit/1(u)

== system gm_ZynqBF_2tx_fpga/channel_estimator/peakdetect_ch2/correlator2/rx_ram_i_instance28/get_bit ==
  u : Inport  OutDataTypeStr=fixdt(0, 64, 0)  PortDimensions=1  SampleTime=1.86011904761905e-08
  ind : Inport  Port=2  OutDataTypeStr=fixdt(0, 9, 0)  PortDimensions=1  SampleTime=1.86011904761905e-08
  get_bit : MATLAB Function  TreatAsAtomicUnit=on
  y : Outport
  wires:
  get_bit/1(y) -> y/1
  ind/1 -> get_bit/2(ind)
  u/1 -> get_bit/1(u)

== system gm_ZynqBF_2tx_fpga/channel_estimator/peakdetect_ch2/correlator2/rx_ram_i_instance29/get_bit ==
  u : Inport  OutDataTypeStr=fixdt(0, 64, 0)  PortDimensions=1  SampleTime=1.86011904761905e-08
  ind : Inport  Port=2  OutDataTypeStr=fixdt(0, 9, 0)  PortDimensions=1  SampleTime=1.86011904761905e-08
  get_bit : MATLAB Function  TreatAsAtomicUnit=on
  y : Outport
  wires:
  get_bit/1(y) -> y/1
  ind/1 -> get_bit/2(ind)
  u/1 -> get_bit/1(u)

== system gm_ZynqBF_2tx_fpga/channel_estimator/peakdetect_ch2/correlator2/rx_ram_i_instance3/get_bit ==
  u : Inport  OutDataTypeStr=fixdt(0, 64, 0)  PortDimensions=1  SampleTime=1.86011904761905e-08
  ind : Inport  Port=2  OutDataTypeStr=fixdt(0, 9, 0)  PortDimensions=1  SampleTime=1.86011904761905e-08
  get_bit : MATLAB Function  TreatAsAtomicUnit=on
  y : Outport
  wires:
  get_bit/1(y) -> y/1
  ind/1 -> get_bit/2(ind)
  u/1 -> get_bit/1(u)

== system gm_ZynqBF_2tx_fpga/channel_estimator/peakdetect_ch2/correlator2/rx_ram_i_instance30/get_bit ==
  u : Inport  OutDataTypeStr=fixdt(0, 64, 0)  PortDimensions=1  SampleTime=1.86011904761905e-08
  ind : Inport  Port=2  OutDataTypeStr=fixdt(0, 9, 0)  PortDimensions=1  SampleTime=1.86011904761905e-08
  get_bit : MATLAB Function  TreatAsAtomicUnit=on
  y : Outport
  wires:
  get_bit/1(y) -> y/1
  ind/1 -> get_bit/2(ind)
  u/1 -> get_bit/1(u)

== system gm_ZynqBF_2tx_fpga/channel_estimator/peakdetect_ch2/correlator2/rx_ram_i_instance31/get_bit ==
  u : Inport  OutDataTypeStr=fixdt(0, 64, 0)  PortDimensions=1  SampleTime=1.86011904761905e-08
  ind : Inport  Port=2  OutDataTypeStr=fixdt(0, 9, 0)  PortDimensions=1  SampleTime=1.86011904761905e-08
  get_bit : MATLAB Function  TreatAsAtomicUnit=on
  y : Outport
  wires:
  get_bit/1(y) -> y/1
  ind/1 -> get_bit/2(ind)
  u/1 -> get_bit/1(u)

== system gm_ZynqBF_2tx_fpga/channel_estimator/peakdetect_ch2/correlator2/rx_ram_i_instance32/get_bit ==
  u : Inport  OutDataTypeStr=fixdt(0, 64, 0)  PortDimensions=1  SampleTime=1.86011904761905e-08
  ind : Inport  Port=2  OutDataTypeStr=fixdt(0, 9, 0)  PortDimensions=1  SampleTime=1.86011904761905e-08
  get_bit : MATLAB Function  TreatAsAtomicUnit=on
  y : Outport
  wires:
  get_bit/1(y) -> y/1
  ind/1 -> get_bit/2(ind)
  u/1 -> get_bit/1(u)

== system gm_ZynqBF_2tx_fpga/channel_estimator/peakdetect_ch2/correlator2/rx_ram_i_instance33/get_bit ==
  u : Inport  OutDataTypeStr=fixdt(0, 64, 0)  PortDimensions=1  SampleTime=1.86011904761905e-08
  ind : Inport  Port=2  OutDataTypeStr=fixdt(0, 9, 0)  PortDimensions=1  SampleTime=1.86011904761905e-08
  get_bit : MATLAB Function  TreatAsAtomicUnit=on
  y : Outport
  wires:
  get_bit/1(y) -> y/1
  ind/1 -> get_bit/2(ind)
  u/1 -> get_bit/1(u)

== system gm_ZynqBF_2tx_fpga/channel_estimator/peakdetect_ch2/correlator2/rx_ram_i_instance34/get_bit ==
  u : Inport  OutDataTypeStr=fixdt(0, 64, 0)  PortDimensions=1  SampleTime=1.86011904761905e-08
  ind : Inport  Port=2  OutDataTypeStr=fixdt(0, 9, 0)  PortDimensions=1  SampleTime=1.86011904761905e-08
  get_bit : MATLAB Function  TreatAsAtomicUnit=on
  y : Outport
  wires:
  get_bit/1(y) -> y/1
  ind/1 -> get_bit/2(ind)
  u/1 -> get_bit/1(u)

== system gm_ZynqBF_2tx_fpga/channel_estimator/peakdetect_ch2/correlator2/rx_ram_i_instance35/get_bit ==
  u : Inport  OutDataTypeStr=fixdt(0, 64, 0)  PortDimensions=1  SampleTime=1.86011904761905e-08
  ind : Inport  Port=2  OutDataTypeStr=fixdt(0, 9, 0)  PortDimensions=1  SampleTime=1.86011904761905e-08
  get_bit : MATLAB Function  TreatAsAtomicUnit=on
  y : Outport
  wires:
  get_bit/1(y) -> y/1
  ind/1 -> get_bit/2(ind)
  u/1 -> get_bit/1(u)

== system gm_ZynqBF_2tx_fpga/channel_estimator/peakdetect_ch2/correlator2/rx_ram_i_instance36/get_bit ==
  u : Inport  OutDataTypeStr=fixdt(0, 64, 0)  PortDimensions=1  SampleTime=1.86011904761905e-08
  ind : Inport  Port=2  OutDataTypeStr=fixdt(0, 9, 0)  PortDimensions=1  SampleTime=1.86011904761905e-08
  get_bit : MATLAB Function  TreatAsAtomicUnit=on
  y : Outport
  wires:
  get_bit/1(y) -> y/1
  ind/1 -> get_bit/2(ind)
  u/1 -> get_bit/1(u)

== system gm_ZynqBF_2tx_fpga/channel_estimator/peakdetect_ch2/correlator2/rx_ram_i_instance37/get_bit ==
  u : Inport  OutDataTypeStr=fixdt(0, 64, 0)  PortDimensions=1  SampleTime=1.86011904761905e-08
  ind : Inport  Port=2  OutDataTypeStr=fixdt(0, 9, 0)  PortDimensions=1  SampleTime=1.86011904761905e-08
  get_bit : MATLAB Function  TreatAsAtomicUnit=on
  y : Outport
  wires:
  get_bit/1(y) -> y/1
  ind/1 -> get_bit/2(ind)
  u/1 -> get_bit/1(u)

== system gm_ZynqBF_2tx_fpga/channel_estimator/peakdetect_ch2/correlator2/rx_ram_i_instance38/get_bit ==
  u : Inport  OutDataTypeStr=fixdt(0, 64, 0)  PortDimensions=1  SampleTime=1.86011904761905e-08
  ind : Inport  Port=2  OutDataTypeStr=fixdt(0, 9, 0)  PortDimensions=1  SampleTime=1.86011904761905e-08
  get_bit : MATLAB Function  TreatAsAtomicUnit=on
  y : Outport
  wires:
  get_bit/1(y) -> y/1
  ind/1 -> get_bit/2(ind)
  u/1 -> get_bit/1(u)

== system gm_ZynqBF_2tx_fpga/channel_estimator/peakdetect_ch2/correlator2/rx_ram_i_instance39/get_bit ==
  u : Inport  OutDataTypeStr=fixdt(0, 64, 0)  PortDimensions=1  SampleTime=1.86011904761905e-08
  ind : Inport  Port=2  OutDataTypeStr=fixdt(0, 9, 0)  PortDimensions=1  SampleTime=1.86011904761905e-08
  get_bit : MATLAB Function  TreatAsAtomicUnit=on
  y : Outport
  wires:
  get_bit/1(y) -> y/1
  ind/1 -> get_bit/2(ind)
  u/1 -> get_bit/1(u)

== system gm_ZynqBF_2tx_fpga/channel_estimator/peakdetect_ch2/correlator2/rx_ram_i_instance4/get_bit ==
  u : Inport  OutDataTypeStr=fixdt(0, 64, 0)  PortDimensions=1  SampleTime=1.86011904761905e-08
  ind : Inport  Port=2  OutDataTypeStr=fixdt(0, 9, 0)  PortDimensions=1  SampleTime=1.86011904761905e-08
  get_bit : MATLAB Function  TreatAsAtomicUnit=on
  y : Outport
  wires:
  get_bit/1(y) -> y/1
  ind/1 -> get_bit/2(ind)
  u/1 -> get_bit/1(u)

== system gm_ZynqBF_2tx_fpga/channel_estimator/peakdetect_ch2/correlator2/rx_ram_i_instance40/get_bit ==
  u : Inport  OutDataTypeStr=fixdt(0, 64, 0)  PortDimensions=1  SampleTime=1.86011904761905e-08
  ind : Inport  Port=2  OutDataTypeStr=fixdt(0, 9, 0)  PortDimensions=1  SampleTime=1.86011904761905e-08
  get_bit : MATLAB Function  TreatAsAtomicUnit=on
  y : Outport
  wires:
  get_bit/1(y) -> y/1
  ind/1 -> get_bit/2(ind)
  u/1 -> get_bit/1(u)

== system gm_ZynqBF_2tx_fpga/channel_estimator/peakdetect_ch2/correlator2/rx_ram_i_instance41/get_bit ==
  u : Inport  OutDataTypeStr=fixdt(0, 64, 0)  PortDimensions=1  SampleTime=1.86011904761905e-08
  ind : Inport  Port=2  OutDataTypeStr=fixdt(0, 9, 0)  PortDimensions=1  SampleTime=1.86011904761905e-08
  get_bit : MATLAB Function  TreatAsAtomicUnit=on
  y : Outport
  wires:
  get_bit/1(y) -> y/1
  ind/1 -> get_bit/2(ind)
  u/1 -> get_bit/1(u)

== system gm_ZynqBF_2tx_fpga/channel_estimator/peakdetect_ch2/correlator2/rx_ram_i_instance42/get_bit ==
  u : Inport  OutDataTypeStr=fixdt(0, 64, 0)  PortDimensions=1  SampleTime=1.86011904761905e-08
  ind : Inport  Port=2  OutDataTypeStr=fixdt(0, 9, 0)  PortDimensions=1  SampleTime=1.86011904761905e-08
  get_bit : MATLAB Function  TreatAsAtomicUnit=on
  y : Outport
  wires:
  get_bit/1(y) -> y/1
  ind/1 -> get_bit/2(ind)
  u/1 -> get_bit/1(u)

== system gm_ZynqBF_2tx_fpga/channel_estimator/peakdetect_ch2/correlator2/rx_ram_i_instance43/get_bit ==
  u : Inport  OutDataTypeStr=fixdt(0, 64, 0)  PortDimensions=1  SampleTime=1.86011904761905e-08
  ind : Inport  Port=2  OutDataTypeStr=fixdt(0, 9, 0)  PortDimensions=1  SampleTime=1.86011904761905e-08
  get_bit : MATLAB Function  TreatAsAtomicUnit=on
  y : Outport
  wires:
  get_bit/1(y) -> y/1
  ind/1 -> get_bit/2(ind)
  u/1 -> get_bit/1(u)

== system gm_ZynqBF_2tx_fpga/channel_estimator/peakdetect_ch2/correlator2/rx_ram_i_instance44/get_bit ==
  u : Inport  OutDataTypeStr=fixdt(0, 64, 0)  PortDimensions=1  SampleTime=1.86011904761905e-08
  ind : Inport  Port=2  OutDataTypeStr=fixdt(0, 9, 0)  PortDimensions=1  SampleTime=1.86011904761905e-08
  get_bit : MATLAB Function  TreatAsAtomicUnit=on
  y : Outport
  wires:
  get_bit/1(y) -> y/1
  ind/1 -> get_bit/2(ind)
  u/1 -> get_bit/1(u)

== system gm_ZynqBF_2tx_fpga/channel_estimator/peakdetect_ch2/correlator2/rx_ram_i_instance45/get_bit ==
  u : Inport  OutDataTypeStr=fixdt(0, 64, 0)  PortDimensions=1  SampleTime=1.86011904761905e-08
  ind : Inport  Port=2  OutDataTypeStr=fixdt(0, 9, 0)  PortDimensions=1  SampleTime=1.86011904761905e-08
  get_bit : MATLAB Function  TreatAsAtomicUnit=on
  y : Outport
  wires:
  get_bit/1(y) -> y/1
  ind/1 -> get_bit/2(ind)
  u/1 -> get_bit/1(u)

== system gm_ZynqBF_2tx_fpga/channel_estimator/peakdetect_ch2/correlator2/rx_ram_i_instance46/get_bit ==
  u : Inport  OutDataTypeStr=fixdt(0, 64, 0)  PortDimensions=1  SampleTime=1.86011904761905e-08
  ind : Inport  Port=2  OutDataTypeStr=fixdt(0, 9, 0)  PortDimensions=1  SampleTime=1.86011904761905e-08
  get_bit : MATLAB Function  TreatAsAtomicUnit=on
  y : Outport
  wires:
  get_bit/1(y) -> y/1
  ind/1 -> get_bit/2(ind)
  u/1 -> get_bit/1(u)

== system gm_ZynqBF_2tx_fpga/channel_estimator/peakdetect_ch2/correlator2/rx_ram_i_instance47/get_bit ==
  u : Inport  OutDataTypeStr=fixdt(0, 64, 0)  PortDimensions=1  SampleTime=1.86011904761905e-08
  ind : Inport  Port=2  OutDataTypeStr=fixdt(0, 9, 0)  PortDimensions=1  SampleTime=1.86011904761905e-08
  get_bit : MATLAB Function  TreatAsAtomicUnit=on
  y : Outport
  wires:
  get_bit/1(y) -> y/1
  ind/1 -> get_bit/2(ind)
  u/1 -> get_bit/1(u)

== system gm_ZynqBF_2tx_fpga/channel_estimator/peakdetect_ch2/correlator2/rx_ram_i_instance48/get_bit ==
  u : Inport  OutDataTypeStr=fixdt(0, 64, 0)  PortDimensions=1  SampleTime=1.86011904761905e-08
  ind : Inport  Port=2  OutDataTypeStr=fixdt(0, 9, 0)  PortDimensions=1  SampleTime=1.86011904761905e-08
  get_bit : MATLAB Function  TreatAsAtomicUnit=on
  y : Outport
  wires:
  get_bit/1(y) -> y/1
  ind/1 -> get_bit/2(ind)
  u/1 -> get_bit/1(u)

== system gm_ZynqBF_2tx_fpga/channel_estimator/peakdetect_ch2/correlator2/rx_ram_i_instance49/get_bit ==
  u : Inport  OutDataTypeStr=fixdt(0, 64, 0)  PortDimensions=1  SampleTime=1.86011904761905e-08
  ind : Inport  Port=2  OutDataTypeStr=fixdt(0, 9, 0)  PortDimensions=1  SampleTime=1.86011904761905e-08
  get_bit : MATLAB Function  TreatAsAtomicUnit=on
  y : Outport
  wires:
  get_bit/1(y) -> y/1
  ind/1 -> get_bit/2(ind)
  u/1 -> get_bit/1(u)

== system gm_ZynqBF_2tx_fpga/channel_estimator/peakdetect_ch2/correlator2/rx_ram_i_instance5/get_bit ==
  u : Inport  OutDataTypeStr=fixdt(0, 64, 0)  PortDimensions=1  SampleTime=1.86011904761905e-08
  ind : Inport  Port=2  OutDataTypeStr=fixdt(0, 9, 0)  PortDimensions=1  SampleTime=1.86011904761905e-08
  get_bit : MATLAB Function  TreatAsAtomicUnit=on
  y : Outport
  wires:
  get_bit/1(y) -> y/1
  ind/1 -> get_bit/2(ind)
  u/1 -> get_bit/1(u)

== system gm_ZynqBF_2tx_fpga/channel_estimator/peakdetect_ch2/correlator2/rx_ram_i_instance50/get_bit ==
  u : Inport  OutDataTypeStr=fixdt(0, 64, 0)  PortDimensions=1  SampleTime=1.86011904761905e-08
  ind : Inport  Port=2  OutDataTypeStr=fixdt(0, 9, 0)  PortDimensions=1  SampleTime=1.86011904761905e-08
  get_bit : MATLAB Function  TreatAsAtomicUnit=on
  y : Outport
  wires:
  get_bit/1(y) -> y/1
  ind/1 -> get_bit/2(ind)
  u/1 -> get_bit/1(u)

== system gm_ZynqBF_2tx_fpga/channel_estimator/peakdetect_ch2/correlator2/rx_ram_i_instance51/get_bit ==
  u : Inport  OutDataTypeStr=fixdt(0, 64, 0)  PortDimensions=1  SampleTime=1.86011904761905e-08
  ind : Inport  Port=2  OutDataTypeStr=fixdt(0, 9, 0)  PortDimensions=1  SampleTime=1.86011904761905e-08
  get_bit : MATLAB Function  TreatAsAtomicUnit=on
  y : Outport
  wires:
  get_bit/1(y) -> y/1
  ind/1 -> get_bit/2(ind)
  u/1 -> get_bit/1(u)

== system gm_ZynqBF_2tx_fpga/channel_estimator/peakdetect_ch2/correlator2/rx_ram_i_instance52/get_bit ==
  u : Inport  OutDataTypeStr=fixdt(0, 64, 0)  PortDimensions=1  SampleTime=1.86011904761905e-08
  ind : Inport  Port=2  OutDataTypeStr=fixdt(0, 9, 0)  PortDimensions=1  SampleTime=1.86011904761905e-08
  get_bit : MATLAB Function  TreatAsAtomicUnit=on
  y : Outport
  wires:
  get_bit/1(y) -> y/1
  ind/1 -> get_bit/2(ind)
  u/1 -> get_bit/1(u)

== system gm_ZynqBF_2tx_fpga/channel_estimator/peakdetect_ch2/correlator2/rx_ram_i_instance53/get_bit ==
  u : Inport  OutDataTypeStr=fixdt(0, 64, 0)  PortDimensions=1  SampleTime=1.86011904761905e-08
  ind : Inport  Port=2  OutDataTypeStr=fixdt(0, 9, 0)  PortDimensions=1  SampleTime=1.86011904761905e-08
  get_bit : MATLAB Function  TreatAsAtomicUnit=on
  y : Outport
  wires:
  get_bit/1(y) -> y/1
  ind/1 -> get_bit/2(ind)
  u/1 -> get_bit/1(u)

== system gm_ZynqBF_2tx_fpga/channel_estimator/peakdetect_ch2/correlator2/rx_ram_i_instance54/get_bit ==
  u : Inport  OutDataTypeStr=fixdt(0, 64, 0)  PortDimensions=1  SampleTime=1.86011904761905e-08
  ind : Inport  Port=2  OutDataTypeStr=fixdt(0, 9, 0)  PortDimensions=1  SampleTime=1.86011904761905e-08
  get_bit : MATLAB Function  TreatAsAtomicUnit=on
  y : Outport
  wires:
  get_bit/1(y) -> y/1
  ind/1 -> get_bit/2(ind)
  u/1 -> get_bit/1(u)

== system gm_ZynqBF_2tx_fpga/channel_estimator/peakdetect_ch2/correlator2/rx_ram_i_instance55/get_bit ==
  u : Inport  OutDataTypeStr=fixdt(0, 64, 0)  PortDimensions=1  SampleTime=1.86011904761905e-08
  ind : Inport  Port=2  OutDataTypeStr=fixdt(0, 9, 0)  PortDimensions=1  SampleTime=1.86011904761905e-08
  get_bit : MATLAB Function  TreatAsAtomicUnit=on
  y : Outport
  wires:
  get_bit/1(y) -> y/1
  ind/1 -> get_bit/2(ind)
  u/1 -> get_bit/1(u)

== system gm_ZynqBF_2tx_fpga/channel_estimator/peakdetect_ch2/correlator2/rx_ram_i_instance56/get_bit ==
  u : Inport  OutDataTypeStr=fixdt(0, 64, 0)  PortDimensions=1  SampleTime=1.86011904761905e-08
  ind : Inport  Port=2  OutDataTypeStr=fixdt(0, 9, 0)  PortDimensions=1  SampleTime=1.86011904761905e-08
  get_bit : MATLAB Function  TreatAsAtomicUnit=on
  y : Outport
  wires:
  get_bit/1(y) -> y/1
  ind/1 -> get_bit/2(ind)
  u/1 -> get_bit/1(u)

== system gm_ZynqBF_2tx_fpga/channel_estimator/peakdetect_ch2/correlator2/rx_ram_i_instance57/get_bit ==
  u : Inport  OutDataTypeStr=fixdt(0, 64, 0)  PortDimensions=1  SampleTime=1.86011904761905e-08
  ind : Inport  Port=2  OutDataTypeStr=fixdt(0, 9, 0)  PortDimensions=1  SampleTime=1.86011904761905e-08
  get_bit : MATLAB Function  TreatAsAtomicUnit=on
  y : Outport
  wires:
  get_bit/1(y) -> y/1
  ind/1 -> get_bit/2(ind)
  u/1 -> get_bit/1(u)

== system gm_ZynqBF_2tx_fpga/channel_estimator/peakdetect_ch2/correlator2/rx_ram_i_instance58/get_bit ==
  u : Inport  OutDataTypeStr=fixdt(0, 64, 0)  PortDimensions=1  SampleTime=1.86011904761905e-08
  ind : Inport  Port=2  OutDataTypeStr=fixdt(0, 9, 0)  PortDimensions=1  SampleTime=1.86011904761905e-08
  get_bit : MATLAB Function  TreatAsAtomicUnit=on
  y : Outport
  wires:
  get_bit/1(y) -> y/1
  ind/1 -> get_bit/2(ind)
  u/1 -> get_bit/1(u)

== system gm_ZynqBF_2tx_fpga/channel_estimator/peakdetect_ch2/correlator2/rx_ram_i_instance59/get_bit ==
  u : Inport  OutDataTypeStr=fixdt(0, 64, 0)  PortDimensions=1  SampleTime=1.86011904761905e-08
  ind : Inport  Port=2  OutDataTypeStr=fixdt(0, 9, 0)  PortDimensions=1  SampleTime=1.86011904761905e-08
  get_bit : MATLAB Function  TreatAsAtomicUnit=on
  y : Outport
  wires:
  get_bit/1(y) -> y/1
  ind/1 -> get_bit/2(ind)
  u/1 -> get_bit/1(u)

== system gm_ZynqBF_2tx_fpga/channel_estimator/peakdetect_ch2/correlator2/rx_ram_i_instance6/get_bit ==
  u : Inport  OutDataTypeStr=fixdt(0, 64, 0)  PortDimensions=1  SampleTime=1.86011904761905e-08
  ind : Inport  Port=2  OutDataTypeStr=fixdt(0, 9, 0)  PortDimensions=1  SampleTime=1.86011904761905e-08
  get_bit : MATLAB Function  TreatAsAtomicUnit=on
  y : Outport
  wires:
  get_bit/1(y) -> y/1
  ind/1 -> get_bit/2(ind)
  u/1 -> get_bit/1(u)

== system gm_ZynqBF_2tx_fpga/channel_estimator/peakdetect_ch2/correlator2/rx_ram_i_instance60/get_bit ==
  u : Inport  OutDataTypeStr=fixdt(0, 64, 0)  PortDimensions=1  SampleTime=1.86011904761905e-08
  ind : Inport  Port=2  OutDataTypeStr=fixdt(0, 9, 0)  PortDimensions=1  SampleTime=1.86011904761905e-08
  get_bit : MATLAB Function  TreatAsAtomicUnit=on
  y : Outport
  wires:
  get_bit/1(y) -> y/1
  ind/1 -> get_bit/2(ind)
  u/1 -> get_bit/1(u)

== system gm_ZynqBF_2tx_fpga/channel_estimator/peakdetect_ch2/correlator2/rx_ram_i_instance61/get_bit ==
  u : Inport  OutDataTypeStr=fixdt(0, 64, 0)  PortDimensions=1  SampleTime=1.86011904761905e-08
  ind : Inport  Port=2  OutDataTypeStr=fixdt(0, 9, 0)  PortDimensions=1  SampleTime=1.86011904761905e-08
  get_bit : MATLAB Function  TreatAsAtomicUnit=on
  y : Outport
  wires:
  get_bit/1(y) -> y/1
  ind/1 -> get_bit/2(ind)
  u/1 -> get_bit/1(u)

== system gm_ZynqBF_2tx_fpga/channel_estimator/peakdetect_ch2/correlator2/rx_ram_i_instance62/get_bit ==
  u : Inport  OutDataTypeStr=fixdt(0, 64, 0)  PortDimensions=1  SampleTime=1.86011904761905e-08
  ind : Inport  Port=2  OutDataTypeStr=fixdt(0, 9, 0)  PortDimensions=1  SampleTime=1.86011904761905e-08
  get_bit : MATLAB Function  TreatAsAtomicUnit=on
  y : Outport
  wires:
  get_bit/1(y) -> y/1
  ind/1 -> get_bit/2(ind)
  u/1 -> get_bit/1(u)
